simulink model "PD_trajectory_controller_for_FOIPTD_parametric"  (R2019b)
settings: Solver=FixedStepAuto  StartTime=0.0  StopTime=t_final  FixedStep=0.001  MaxStep=1e-3  RelTol=1e-3  EnableMultiTasking=on
undefined symbols (not defined in the file or in its folder): D, D_inner, I, I_inner, K, K_inner, original_poly_x, P, P_inner, poly_x, T1, T1_inner, T2_inner, tau, tau_inner
libraries: simulink x1
settings Model: SimulationMode=accelerator  Creator=msa  LastModifiedBy=aaa_b
settings DataIOCC: SaveFormat=Array  DSMLogging=off  ReturnWorkspaceOutputs=off
settings OptimizationCC: LifeSpan=inf
settings DebuggingCC: SolverPrmCheckMsg=warning  SFUnexpectedBacktrackingDiag=warning  SFNoUnconditionalDefaultTransitionDiag=warning  SFExecutionAtInitializationDiag=none  ArithmeticOperatorsInVariantConditions=warning
settings HardwareCC: ProdBitPerPointer=32  ProdBitPerSizeT=32  ProdBitPerPtrDiffT=32  ProdLargestAtomicFloat=None  ProdIntDivRoundTo=Undefined  ProdEndianess=Unspecified  ProdWordSize=32  ProdHWDeviceType=32-bit Generic
settings ModelReferenceCC: PropagateSignalLabelsOutOfModel=off
settings SFSimCC: SimUseLocalCustomCode=off  CustomCodeUndefinedFunction=UseInterfaceOnly
settings RTWCC: RTWUseLocalCustomCode=off
settings CodeAppCC: StateflowObjectComments=on
settings GRTTargetCC: TargetLangStandard=C89/C90 (ANSI)  GeneratePreprocessorConditionals=Disable all
settings ConfigComp: CovMetricSettings=dw  CovHtmlReporting=on  CovSaveCumulativeToWorkspaceVar=on  CovSaveSingleToWorkspaceVar=on  CovExternalEMLEnable=off  CovSFcnEnable=off

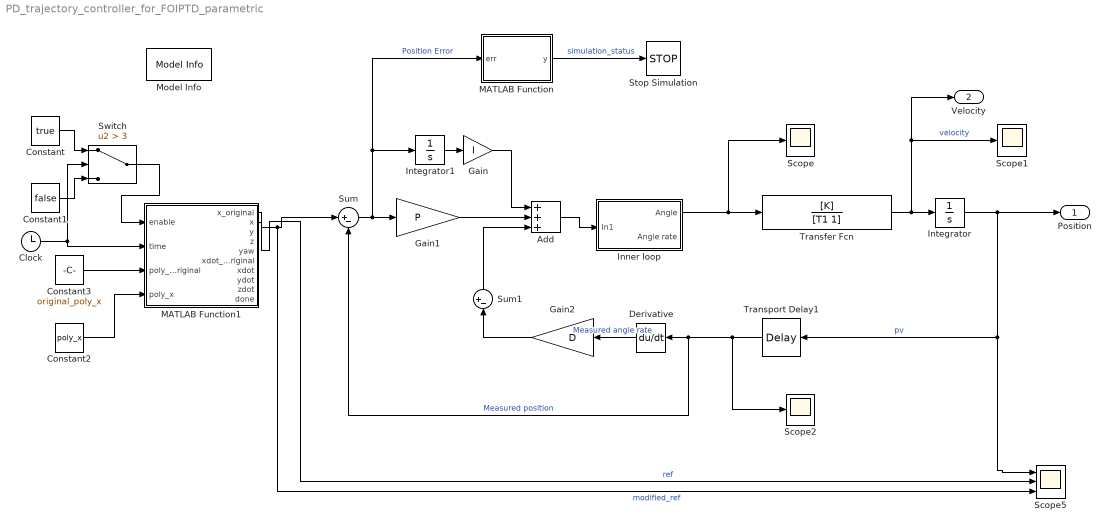
== system PD_trajectory_controller_for_FOIPTD_parametric ==
  Add : Sum  Inputs=+++
  Clock : Clock
  Constant : Constant  Value=true
  Constant1 : Constant  Value=false
  Constant2 : Constant  Value=poly_x
  Constant3 : Constant  Value=original_poly_x
  Derivative : Derivative
  Gain : Gain  Gain=I
  Gain1 : Gain  Gain=P
  Gain2 : Gain  Gain=D
  "Inner loop " : Subsystem
  Integrator : Integrator
  Integrator1 : Integrator
  MATLAB Function : MATLAB Function  TreatAsAtomicUnit=on
  MATLAB Function1 : MATLAB Function  TreatAsAtomicUnit=on
  Model Info : simulink/Model-Wide Utilities/Model Info  Frame=on  DisplayStringWithTags=Model Info How should we take sensors reading WITHOUT delay  HorizontalTextAlignment=Center  LeftAlignmentValue=0.5
  Scope : Scope
  Scope1 : Scope
  Scope2 : Scope
  Scope5 : Scope  NumInputPorts=3
  Stop Simulation : Stop
  Sum : Sum  Inputs=|+-
  Sum1 : Sum  Inputs=+-|
  Switch : Switch  Criteria=u2 > Threshold  Threshold=3
  Transfer Fcn : TransferFcn  Numerator=[K]  Denominator=[T1 1]
  Transport Delay1 : TransportDelay  DelayTime=tau
  "Position " : Outport
  "Velocity " : Outport  Port=2
  wires:
  Integrator1/1 -> Gain/1
  Transfer Fcn/1 -> Scope1/1, "Velocity "/1, Integrator/1  "velocity"
  Gain/1 -> Add/1
  Gain1/1 -> Add/2
  Derivative/1 -> Gain2/1  "Measured angle rate"
  Integrator/1 -> "Position "/1, Scope5/1, Transport Delay1/1  "pv"
  Add/1 -> "Inner loop "/1(In1)
  MATLAB Function/1(y) -> Stop Simulation/1  "simulation_status"
  Sum/1 -> MATLAB Function/1(err), Integrator1/1, Gain1/1  "Position Error"
  Transport Delay1/1 -> Scope2/1, Sum/2, Derivative/1  "Measured position"
  "Inner loop "/1("Angle ") -> Scope/1, Transfer Fcn/1
  Clock/1 -> Switch/2, MATLAB Function1/2(time)
  Switch/1 -> MATLAB Function1/1(enable)
  Constant1/1 -> Switch/3
  Constant/1 -> Switch/1
  MATLAB Function1/2(x) -> Scope5/3, Sum/1  "modified_ref"
  Constant3/1 -> MATLAB Function1/3(poly_x_original)
  MATLAB Function1/1(x_original) -> Scope5/2  "ref"
  Gain2/1 -> Sum1/2
  Sum1/1 -> Add/3
  Constant2/1 -> MATLAB Function1/4(poly_x)

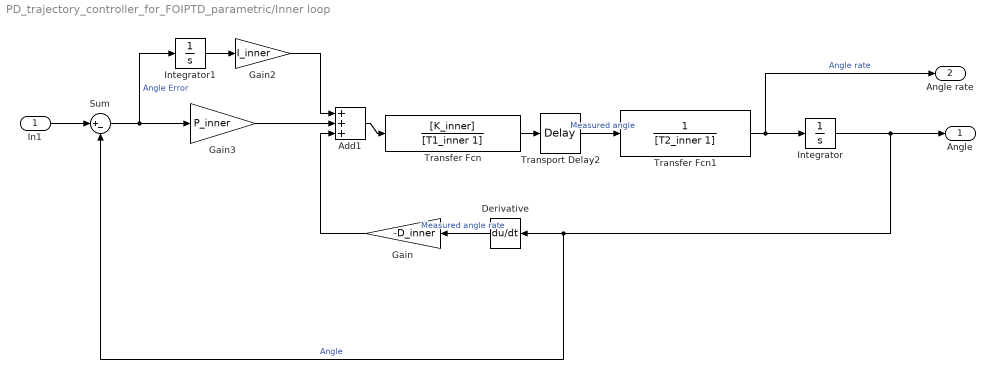
== system PD_trajectory_controller_for_FOIPTD_parametric/Inner loop  ==
  In1 : Inport
  Add1 : Sum  Inputs=+++
  Derivative : Derivative
  Gain : Gain  Gain=-D_inner
  Gain2 : Gain  Gain=I_inner
  Gain3 : Gain  Gain=P_inner
  Integrator : Integrator
  Integrator1 : Integrator
  Sum : Sum  Inputs=|+-
  Transfer Fcn : TransferFcn  Numerator=[K_inner]  Denominator=[T1_inner 1]
  Transfer Fcn1 : TransferFcn  Denominator=[T2_inner 1]
  Transport Delay2 : TransportDelay  DelayTime=tau_inner
  "Angle " : Outport
  "Angle rate " : Outport  Port=2
  wires:
  Sum/1 -> Integrator1/1, Gain3/1  "Angle Error"
  Transfer Fcn1/1 -> "Angle rate "/1, Integrator/1  "Angle rate"
  In1/1 -> Sum/1
  Transfer Fcn/1 -> Transport Delay2/1
  Derivative/1 -> Gain/1  "Measured angle rate"
  Add1/1 -> Transfer Fcn/1
  Integrator/1 -> Derivative/1, Sum/2, "Angle "/1  "Angle"
  Gain2/1 -> Add1/1
  Gain3/1 -> Add1/2
  Integrator1/1 -> Gain2/1
  Gain/1 -> Add1/3
  Transport Delay2/1 -> Transfer Fcn1/1  "Measured angle"

== matlab function PD_trajectory_controller_for_FOIPTD_parametric/MATLAB Function1 ==
  settings: updateMethod=DISCRETE
  data: enable input; x_original output; x output; time input; poly_x_original input; y output; z output; yaw output; xdot_original output; xdot output; ydot output; zdot output; done output; poly_x input
function [x_original, x, y, z, yaw, xdot_original, xdot, ydot, zdot, done]= fcn(enable, time, poly_x_original, poly_x)

persistent start_time
%persistent poly_x
persistent poly_y
persistent poly_z
persistent ts
persistent trajectory_segment
persistent n_order

if isempty(start_time) || isempty(trajectory_segment) || ~enable
    start_time = time;
    trajectory_segment = 1;
end

if isempty(poly_x) || isempty(poly_y) || isempty(poly_z) || isempty(ts)
    g = coder.load('aggressive_man.mat');
    %poly_x = g.polys_x;
    poly_y = g.polys_y;
    poly_z = g.polys_z;
    n_order = g.n_order(1);
    ts = g.ts;
end

x_original=0; x = 0; y = 0; z = 0; yaw=0; done=false;
xdot_original = 0; xdot = 0; ydot = 0; zdot = 0; 
if enable
    t = time - start_time;
    if t > ts(end)
        x_original=0; x = 0; y = 0; z = 1; yaw = 0; done = true;
        xdot_original = 0; xdot = 0; ydot = 0; zdot = 0; 
        return;
    elseif t > ts(trajectory_segment + 1)
        trajectory_segment = trajectory_segment + 1;
        %t = ts(trajectory_segment + 1);
    end
    
    poly_x_i_original = poly_x_original(:, trajectory_segment);
    poly_x_i = poly_x(:, trajectory_segment);
    poly_y_i = poly_y{trajectory_segment};
    poly_z_i = poly_z{trajectory_segment};

    for i=0:n_order
        x_original = x_original + poly_x_i_original(i+1) * t^i;
        y = y + poly_y_i(i+1) * t^i;
        z = z + poly_z_i(i+1) * t^i;
        if i>0
            xdot_original = xdot_original + i * poly_x_i_original(i+1) * t^(i-1);
            ydot = ydot + i * poly_y_i(i+1) * t^(i-1);
            zdot = zdot + i * poly_z_i(i+1) * t^(i-1);
        end
    end
    for i=0:length(poly_x_i)-1        
        x = x + poly_x_i(i+1) * t^i;
        if i>0
            xdot = xdot + i * poly_x_i(i+1) * t^(i-1);
        end
    end
    
end

== matlab function PD_trajectory_controller_for_FOIPTD_parametric/MATLAB Function ==
  data: err input; y output
function y = fcn(err)
if (abs(err)>1000)
    y=1;
else
    y=0;
end
